simulink model "simulink_model"  (R2022a)
settings: Solver=VariableStepAuto  StartTime=0.0  StopTime=10.0  RelTol=1e-3
undefined symbols (not defined in the file): denom, Gd_denom, Gd_num, Gi_denom, Gi_num, Kp, num
settings Model: Creator=Alonso  LastModifiedBy=Alonso

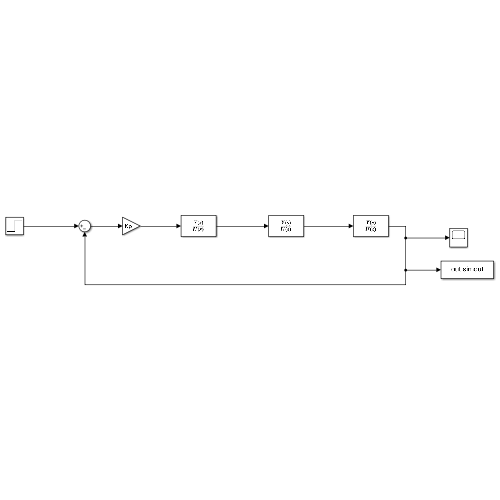
[thumbnail: Simulink's stored preview of the top-level diagram]
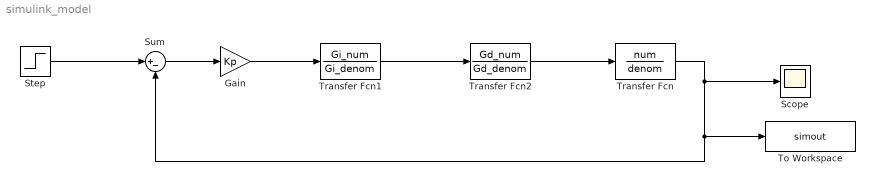
== system simulink_model ==
  Gain : Gain  Gain=Kp
  Scope : Scope
  Step : Step  Time=0.1  After=0.5  SampleTime=0
  Sum : Sum  Inputs=|+-
  To Workspace : ToWorkspace  VariableName=simout  SaveFormat=Timeseries  SampleTime=-1
  Transfer Fcn : TransferFcn  Numerator=num  Denominator=denom
  Transfer Fcn1 : TransferFcn  Numerator=Gi_num  Denominator=Gi_denom
  Transfer Fcn2 : TransferFcn  Numerator=Gd_num  Denominator=Gd_denom
  wires:
  Step/1 -> Sum/1
  Sum/1 -> Gain/1
  Gain/1 -> Transfer Fcn1/1
  Transfer Fcn2/1 -> Transfer Fcn/1
  Transfer Fcn/1 -> Scope/1, To Workspace/1, Sum/2
  Transfer Fcn1/1 -> Transfer Fcn2/1
